simulink model "BEVController_harness_model"  (R2024b)
settings: Solver=VariableStepAuto  StartTime=0.0  StopTime=1000  RelTol=1e-3  AbsTol=1e-3
PreLoadFcn:
  | BEVController_harness_setup
undefined symbols (not defined in the file): bevControl
libraries: simulink x1
settings Model: Creator=isaacito  LastModifiedBy=isaacito
settings SolverCC: AutoScaleAbsTol=off  AlgebraicLoopSolver=TrustRegion
settings DataIOCC: DSMLogging=off
settings OptimizationCC: ReuseModelBlockBuffer=off
settings DebuggingCC: UnconnectedInputMsg=warning  UnconnectedOutputMsg=warning  UnconnectedLineMsg=warning
settings ModelReferenceCC: EnableRefExpFcnMdlSchedulingChecks=on
settings RTWCC: GPUComputeCapability=3.5  DLArmComputeVersion=19.05
settings SimscapeCC: SimscapeLogType=all  SimscapeLogSimulationStatistics=on  SimscapeLogLimitData=off

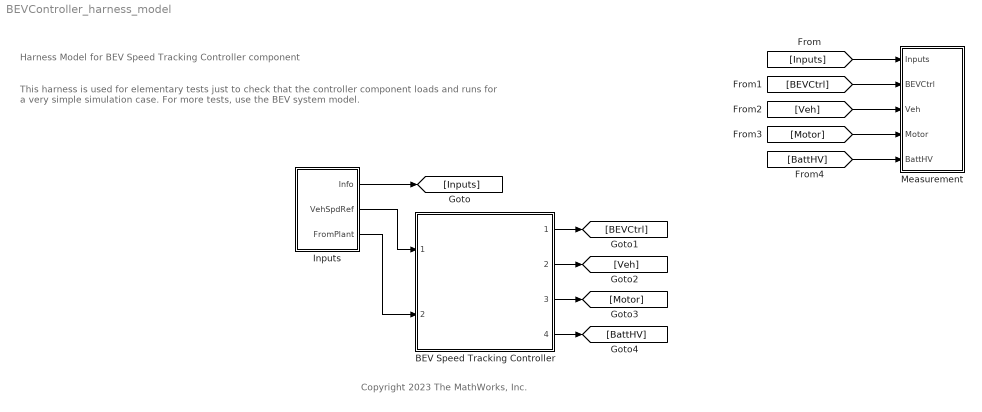
== system BEVController_harness_model ==
  note: This harness is used for elementary tests
      | just to check that the controller component loads and runs
      | for a very simple simulation case.
      | For more tests, use the BEV system model.
  note: Harness Model for BEV Speed Tracking Controller component
  note: Copyright 2023 The MathWorks, Inc.
  BEV Speed Tracking Controller : Subsystem  ReferencedSubsystem=BEVController_refsub_Basic
      settings: OpenFcn=|
      | % Look under mask:
      | open_system(gcb, "force")
  Inputs : Subsystem
  Measurement : Subsystem
  wires:
  Inputs/2(VehSpdRef) -> BEV Speed Tracking Controller/1
  Inputs/3(FromPlant) -> BEV Speed Tracking Controller/2
  Inputs/1(Info) -> [Inputs]
  BEV Speed Tracking Controller/1 -> [BEVCtrl]
  BEV Speed Tracking Controller/2 -> [Veh]
  BEV Speed Tracking Controller/3 -> [Motor]
  BEV Speed Tracking Controller/4 -> [BattHV]
  [Inputs] -> Measurement/1(Inputs)
  [BEVCtrl] -> Measurement/2(BEVCtrl)
  [Veh] -> Measurement/3(Veh)
  [Motor] -> Measurement/4(Motor)
  [BattHV] -> Measurement/5(BattHV)

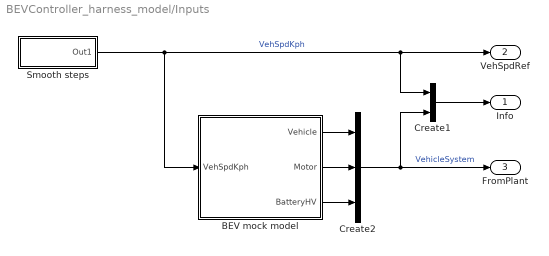
== system BEVController_harness_model/Inputs ==
  BEV mock model : Subsystem
  Create1 : BusCreator  Inputs=2
  Create2 : BusCreator  Inputs=3
  Smooth steps : Subsystem  mask(Continuous Multi-Step Signal){dataPoints=[0 200 0; 210 400 10; 410 600 00; 610 800 30; 810 1000 60], deltaT=0.2}
      mask prompts: dataPoints "Data points"; deltaT "Interpolation step [s]"
      mask help:
      | This block generates a signal consisting of smoothly connected flat segments. Data points parameter takes an N-by-3 matrix where each row specifies a flat segment. First column and second column define start and end time of the segment, respectively. Third column defines the value of the segment. Second column can also be NaN to define a point value. Flat segments and point values are smoothly interpolated by Akima spline with the specified interpolation step.
      |
      | For example, a matrix [0 1 5; 3 nan 9; 6 8 7] for Data points defines a signal as follows. First row defines a flat segment from t=0 to t=1 of value 5. Second row defines a point at t=3 of value 9. Third row defines a flat segment from t=6 to t=8 of value 7.
      mask init:
      | sig = SignalDesigner("ContinuousMultiStep");
      | 
      | % Initialization function can access parameter names directly
      | sig.XYData = dataPoints;
      | sig.DeltaX = deltaT;
      | 
      | update(sig)
      mask DialogControl Control3 Prompt: horizontal spacer 1
      mask DialogControl Control4 Prompt: horizontal spacer 2
      mask DialogControl Control5 Prompt: horizontal spacer 3
      mask DialogControl PlotButton Prompt: Plot
      mask DialogControl PlotButton Callback: SignalSourceBlockCallback.plotContinuousMultiStep(gcb);
      mask Display: disp("Continuous" + newline + "Multi-Step")
  Info : Outport
  VehSpdRef : Outport  Port=2
  FromPlant : Outport  Port=3
  wires:
  Create2/1 -> Create1/2, FromPlant/1  "VehicleSystem"
  Create1/1 -> Info/1
  BEV mock model/1(Vehicle) -> Create2/1
  BEV mock model/2(Motor) -> Create2/2
  BEV mock model/3(BatteryHV) -> Create2/3
  Smooth steps/1(Out1) -> BEV mock model/1(VehSpdKph), Create1/1, VehSpdRef/1  "VehSpdKph"

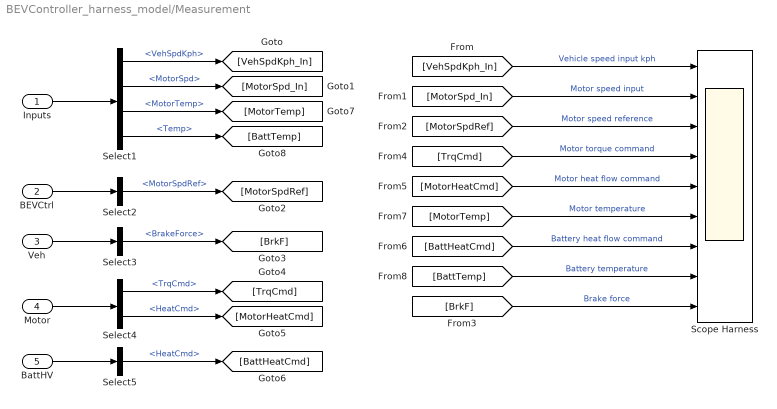
== system BEVController_harness_model/Measurement ==
  Inputs : Inport
  BEVCtrl : Inport  Port=2
  Veh : Inport  Port=3
  Motor : Inport  Port=4
  BattHV : Inport  Port=5
  Scope Harness : Scope  NumInputPorts=9
  Select1 : BusSelector  OutputSignals=VehSpdKph,VehicleSystem.Motor.MotorSpd,VehicleSystem.Motor.MotorTemp,VehicleSystem.Battery.Temp
  Select2 : BusSelector  OutputSignals=MotorSpdRef
  Select3 : BusSelector  OutputSignals=BrakeForce
  Select4 : BusSelector  OutputSignals=TrqCmd,HeatCmd
  Select5 : BusSelector  OutputSignals=HeatCmd
  wires:
  Inputs/1 -> Select1/1
  Select1/1 -> [VehSpdKph_In]  "<VehSpdKph>"
  Select1/2 -> [MotorSpd_In]  "<MotorSpd>"
  BEVCtrl/1 -> Select2/1
  Select2/1 -> [MotorSpdRef]  "<MotorSpdRef>"
  Veh/1 -> Select3/1
  Select3/1 -> [BrkF]  "<BrakeForce>"
  Motor/1 -> Select4/1
  Select4/1 -> [TrqCmd]  "<TrqCmd>"
  Select4/2 -> [MotorHeatCmd]  "<HeatCmd>"
  BattHV/1 -> Select5/1
  Select5/1 -> [BattHeatCmd]  "<HeatCmd>"
  [VehSpdKph_In] -> Scope Harness/1  "Vehicle speed input kph"
  [MotorSpd_In] -> Scope Harness/2  "Motor speed input"
  [MotorSpdRef] -> Scope Harness/3  "Motor speed reference"
  Select1/3 -> [MotorTemp]  "<MotorTemp>"
  Select1/4 -> [BattTemp]  "<Temp>"
  [TrqCmd] -> Scope Harness/4  "Motor torque command"
  [MotorHeatCmd] -> Scope Harness/5  "Motor heat flow command"
  [MotorTemp] -> Scope Harness/6  "Motor temperature"
  [BattHeatCmd] -> Scope Harness/7  "Battery heat flow command"
  [BattTemp] -> Scope Harness/8  "Battery temperature"
  [BrkF] -> Scope Harness/9  "Brake force"

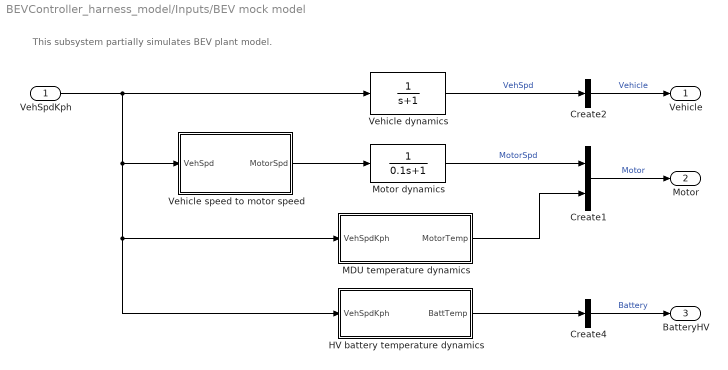
== system BEVController_harness_model/Inputs/BEV mock model ==
  note: This subsystem partially simulates BEV plant model.
  VehSpdKph : Inport
  Create1 : BusCreator  Inputs=2
  Create2 : BusCreator  Inputs=1
  Create4 : BusCreator  Inputs=1
  HV battery temperature dynamics : Subsystem
  MDU temperature dynamics : Subsystem
  Motor dynamics : TransferFcn  Denominator=[0.1 1]
  Vehicle dynamics : TransferFcn  Denominator=[1 1]
  Vehicle speed to motor speed : Subsystem
  Vehicle : Outport
  Motor : Outport  Port=2
  BatteryHV : Outport  Port=3
  wires:
  Vehicle speed to motor speed/1(MotorSpd) -> Motor dynamics/1
  Create2/1 -> Vehicle/1  "Vehicle"
  Motor dynamics/1 -> Create1/1  "MotorSpd"
  Create1/1 -> Motor/1  "Motor"
  Vehicle dynamics/1 -> Create2/1  "VehSpd"
  VehSpdKph/1 -> Vehicle dynamics/1, HV battery temperature dynamics/1(VehSpdKph), MDU temperature dynamics/1(VehSpdKph), Vehicle speed to motor speed/1(VehSpd)
  Create4/1 -> BatteryHV/1  "Battery"
  MDU temperature dynamics/1(MotorTemp) -> Create1/2
  HV battery temperature dynamics/1(BattTemp) -> Create4/1

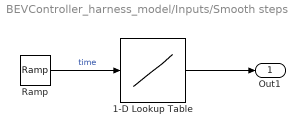
== system BEVController_harness_model/Inputs/Smooth steps ==
  1-D Lookup Table : Lookup_n-D  NumberOfTableDimensions=1  BreakpointsForDimension1=sig.Data.X  Table=sig.Data.Y  InternalRulePriority=Speed  RndMeth=Simplest
  Ramp : simulink/Sources/Ramp  slope=1  start=0  InitialOutput=0
      settings: AttributesFormatString=|
      | Slope: %<slope>
      | Start time: %<start>
      | Initial output: %<InitialOutput>
  Out1 : Outport
  wires:
  1-D Lookup Table/1 -> Out1/1
  Ramp/1 -> 1-D Lookup Table/1  "time"

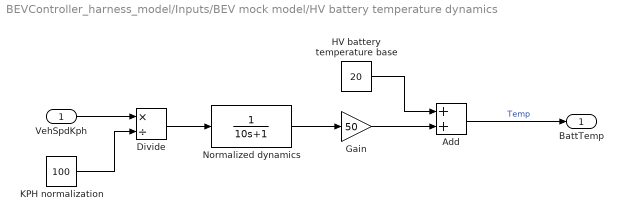
== system BEVController_harness_model/Inputs/BEV mock model/HV battery temperature dynamics ==
  VehSpdKph : Inport  Unit=km/hr
  Add : Sum
  Divide : Product  Inputs=*/
  Gain : Gain  Gain=50
  HV battery temperature base : Constant  Value=20
  KPH normalization : Constant  Value=100
  Normalized dynamics : TransferFcn  Denominator=[10 1]
  BattTemp : Outport  Unit=degC
  wires:
  KPH normalization/1 -> Divide/2
  Add/1 -> BattTemp/1  "Temp"
  Gain/1 -> Add/2
  HV battery temperature base/1 -> Add/1
  Divide/1 -> Normalized dynamics/1
  Normalized dynamics/1 -> Gain/1
  VehSpdKph/1 -> Divide/1

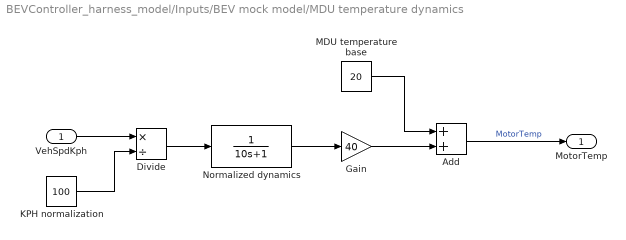
== system BEVController_harness_model/Inputs/BEV mock model/MDU temperature dynamics ==
  VehSpdKph : Inport  Unit=km/hr
  Add : Sum
  Divide : Product  Inputs=*/
  Gain : Gain  Gain=40
  KPH normalization : Constant  Value=100
  MDU temperature base : Constant  Value=20
  Normalized dynamics : TransferFcn  Denominator=[10 1]
  MotorTemp : Outport  Unit=degC
  wires:
  KPH normalization/1 -> Divide/2
  Add/1 -> MotorTemp/1  "MotorTemp"
  Gain/1 -> Add/2
  MDU temperature base/1 -> Add/1
  Divide/1 -> Normalized dynamics/1
  Normalized dynamics/1 -> Gain/1
  VehSpdKph/1 -> Divide/1

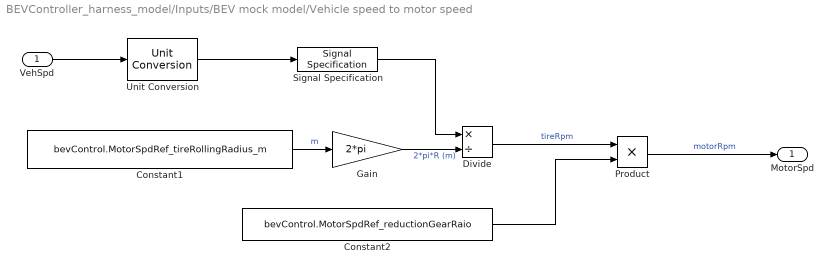
== system BEVController_harness_model/Inputs/BEV mock model/Vehicle speed to motor speed ==
  VehSpd : Inport  Unit=km/hr
  Constant1 : Constant  Value=bevControl.MotorSpdRef_tireRollingRadius_m
  Constant2 : Constant  Value=bevControl.MotorSpdRef_reductionGearRaio
  Divide : Product  Inputs=*/
  Gain : Gain  Gain=2*pi
  Product : Product
  Signal Specification : SignalSpecification  Unit=m/min
  Unit Conversion : UnitConversion
  MotorSpd : Outport  Unit=rpm  VectorParamsAs1DForOutWhenUnconnected=off
  wires:
  Constant1/1 -> Gain/1  "m"
  Product/1 -> MotorSpd/1  "motorRpm"
  Constant2/1 -> Product/2
  Divide/1 -> Product/1  "tireRpm"
  Gain/1 -> Divide/2  "2*pi*R (m)"
  Signal Specification/1 -> Divide/1
  Unit Conversion/1 -> Signal Specification/1
  VehSpd/1 -> Unit Conversion/1
